simulink model "State_Simplified7DOF"  (R2019b)
settings: Solver=VariableStepAuto  StartTime=0.0  StopTime=10.0  RelTol=1e-3
libraries: vehdynlibsteering x1
settings Model: Creator=yeyuan  LastModifiedBy=yeyuan
settings DebuggingCC: ModelReferenceExtraNoncontSigs=warning

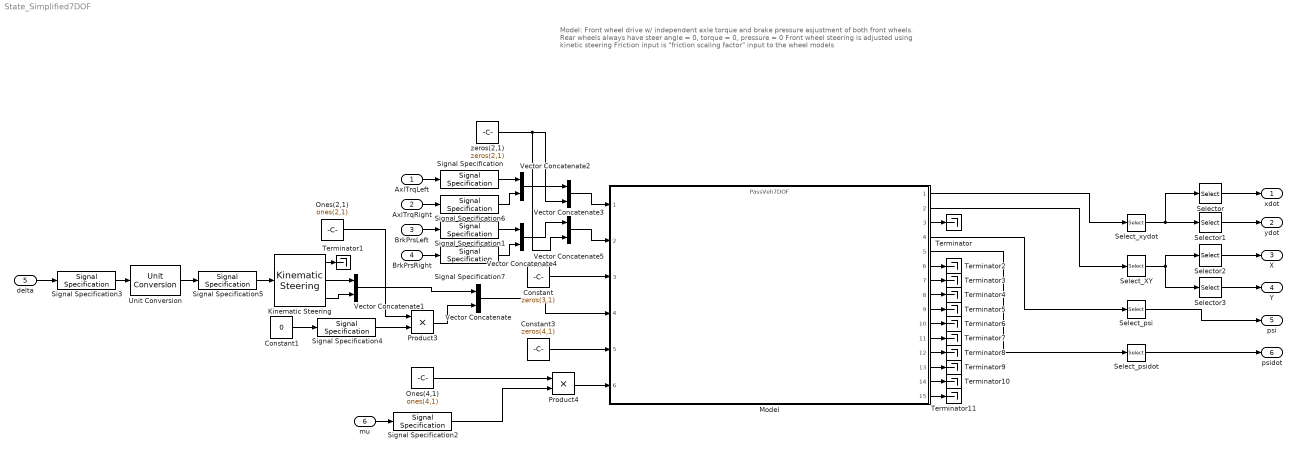
== system State_Simplified7DOF ==
  note: Model:
      | Front wheel drive w/ independent axle torque and brake pressure asjustment of both front wheels.
      | Rear wheels always have steer angle = 0, torque = 0, pressure = 0
      | Front wheel steering is adjusted using kinetic steering
      | Friction input is "friction scaling factor" input to the wheel models
  AxlTrqLeft : Inport
  AxlTrqRight : Inport  Port=2
  BrkPrsLeft : Inport  Port=3
  BrkPrsRight : Inport  Port=4
  delta : Inport  Port=5
  mu : Inport  Port=6
  Constant : Constant  Value=zeros(3,1)
  Constant1 : Constant  Value=0
  Constant3 : Constant  Value=zeros(4,1)
  Kinematic Steering : vehdynlibsteering/Kinematic Steering  StrgType=Ackerman  StrgRatioType=Constant  Loc=Front  NrmlFctr=0.01  TrckWdth=1.922  WhlBase=(1.515+1.504)  Db=0  StrgRng=pi/2  StrgAngBpts="[-6.2832   -5.0265   -3.7699   -2.5133   -1.2566         0    1.2566    2.5133    3.7699    5.0265    6.2832]"  StrgRatioTbl=|  StrgRatio=1  StrgArmLngth=0.1  RckCsLngth=0.5  TieRodLngth=0.248  D=0.2  PnnRadius=0.00085818  PnnRadiusTbl="[0.0055    0.0055    0.0056    0.0057    0.0058    0.0057    0.0057    0.0057    0.0056    0.0055    0.0055]"  RodLngth=0.1  ParaArmLngth=0.9  aMode=2
      | [13.5000   13.3750   13.2500   13.1250   13.0000   13.0000   13.0000   13.1250   13.2500   13.3750   13.5000
      | ]
      settings: SourceProductName=Vehicle Dynamics Blockset
  Model : ModelReference  ModelNameDialog=PassVeh7DOF.slx  SimulationMode=Normal  ModelReferenceVersion=1.147
  Ones(2,1) : Constant  Value=ones(2,1)  OutDataTypeStr=Inherit: Inherit via back propagation
  Ones(4,1) : Constant  Value=ones(4,1)  OutDataTypeStr=Inherit: Inherit via back propagation
  Product3 : Product
  Product4 : Product
  Select_XY : Selector  InputPortWidth=3  IndexOptions=Index vector (dialog)  Indices=[1 2]  OutputSizes=1
  Select_psi : Selector  InputPortWidth=3  IndexOptions=Index vector (dialog)  Indices=[3]  OutputSizes=1
  Select_psidot : Selector  InputPortWidth=3  IndexOptions=Index vector (dialog)  Indices=[3]  OutputSizes=1
  Select_xydot : Selector  InputPortWidth=3  IndexOptions=Index vector (dialog)  Indices=[1 3]  OutputSizes=1
  Selector : Selector  InputPortWidth=2  IndexOptions=Index vector (dialog)  Indices=[1]  OutputSizes=1
  Selector1 : Selector  InputPortWidth=2  IndexOptions=Index vector (dialog)  Indices=[2]  OutputSizes=1
  Selector2 : Selector  InputPortWidth=2  IndexOptions=Index vector (dialog)  Indices=[1]  OutputSizes=1
  Selector3 : Selector  InputPortWidth=2  IndexOptions=Index vector (dialog)  Indices=[2]  OutputSizes=1
  Signal Specification : SignalSpecification  Unit=N*m
  Signal Specification1 : SignalSpecification  Unit=Pa
  Signal Specification2 : SignalSpecification  Unit=1
  Signal Specification3 : SignalSpecification  Unit=deg
  Signal Specification4 : SignalSpecification  Unit=rad
  Signal Specification5 : SignalSpecification  Unit=rad
  Signal Specification6 : SignalSpecification  Unit=N*m
  Signal Specification7 : SignalSpecification  Unit=Pa
  Terminator{,1..11} (12 alike) : Terminator
  Unit Conversion : UnitConversion
  Vector Concatenate{,1..5} (6 alike) : Concatenate
  zeros(2,1) : Constant  Value=zeros(2,1)  OutDataTypeStr=Inherit: Inherit via back propagation
  xdot : Outport
  ydot : Outport  Port=2
  X : Outport  Port=3
  Y : Outport  Port=4
  psi : Outport  Port=5
  psidot : Outport  Port=6
  wires:
  Constant3/1 -> Model/5
  Constant/1 -> Model/3
  mu/1 -> Signal Specification2/1
  AxlTrqLeft/1 -> Signal Specification/1
  BrkPrsLeft/1 -> Signal Specification1/1
  delta/1 -> Signal Specification3/1
  Signal Specification3/1 -> Unit Conversion/1
  Constant1/1 -> Signal Specification4/1
  Unit Conversion/1 -> Signal Specification5/1
  Model/6 -> Terminator2/1
  Model/7 -> Terminator3/1
  Model/8 -> Terminator4/1
  Model/9 -> Terminator5/1
  Model/10 -> Terminator6/1
  Model/11 -> Terminator7/1
  Model/12 -> Terminator8/1
  Model/13 -> Terminator9/1
  Model/14 -> Terminator10/1
  Model/15 -> Terminator11/1
  Ones(2,1)/1 -> Product3/1
  Signal Specification4/1 -> Product3/2
  Product3/1 -> Vector Concatenate/2
  Vector Concatenate/1 -> Model/4
  Product4/1 -> Model/6
  Signal Specification2/1 -> Product4/2
  Model/4 -> Select_psi/1
  Model/5 -> Select_psidot/1
  Model/2 -> Select_XY/1
  Model/1 -> Select_xydot/1
  Select_xydot/1 -> Selector1/1, Selector/1
  Selector/1 -> xdot/1
  Selector1/1 -> ydot/1
  Select_XY/1 -> Selector3/1, Selector2/1
  Selector2/1 -> X/1
  Selector3/1 -> Y/1
  Select_psi/1 -> psi/1
  Select_psidot/1 -> psidot/1
  Model/3 -> Terminator/1
  Signal Specification5/1 -> Kinematic Steering/1
  Kinematic Steering/2 -> Vector Concatenate1/1
  Kinematic Steering/3 -> Vector Concatenate1/2
  Vector Concatenate1/1 -> Vector Concatenate/1
  Kinematic Steering/1 -> Terminator1/1
  AxlTrqRight/1 -> Signal Specification6/1
  Ones(4,1)/1 -> Product4/1
  Signal Specification/1 -> Vector Concatenate2/1
  Signal Specification6/1 -> Vector Concatenate2/2
  Vector Concatenate2/1 -> Vector Concatenate3/1
  zeros(2,1)/1 -> Vector Concatenate5/2, Vector Concatenate3/2
  Vector Concatenate3/1 -> Model/1
  BrkPrsRight/1 -> Signal Specification7/1
  Signal Specification1/1 -> Vector Concatenate4/1
  Signal Specification7/1 -> Vector Concatenate4/2
  Vector Concatenate4/1 -> Vector Concatenate5/1
  Vector Concatenate5/1 -> Model/2
